simulink model "mech_brownian_osc_control"  (Simulink 7.1)
settings: Solver=ode113  StartTime=0.0  StopTime=300  RelTol=1e-4
PreLoadFcn:
  | % Define primitive constants once
  | 
  | k = 1e-7; b = 12*pi*1e-9; m = 1e-7/16/pi^2; r = 5e-6;
  | kB = 1.3806503e-23; T = 290; g = 2*kB*T*b;
  | lambda = 1e-8; Flambda = 2.5e-12;
InitFcn:
  | % Define system constants once per simulation
  | 
  | brownian.spring.stiffness = k;
  | brownian.spring.damping = b;
  | brownian.spring.offset = 0;
  | 
  | brownian.control.limit = lambda /2;
  | brownian.control.force = Flambda;
  | 
  | brownian.particle.mass = m;
  | brownian.particle.inertia = (2/5)*m*r^2*eye(3);
  | 
  | brownian.noise.power = g;
  | brownian.noise.sample = 2*pi*sqrt(m/k)/100;
  | brownian.noise.seed = 54321;
  | 
  | brownian.dynamics.mintime = 0.01;
  | brownian.dynamics.minlength = sqrt(g/2/b/k)/1000;
libraries: mblibv1 x7, simulink x6
Description:
  | Stochastic Microcontroller
  | 
  | Modified Brownian motion: A microparticle oscillates with a linear damped microspring while diffusing by the addition of a random white noise force. A microcontroller applies a control force that tries to keep the particle within predefined limits.
  | 
  | The system is ergodic: Averages are computed as time averages and assumed to be equal to statistical ensemble averages over long times.  Based on a magnetic microtweezer system for biophysics research.
settings Model: Creator=dkennedy  LastModifiedBy=batserve  ExtModeAutoUpdateStatusClock=off
settings DebuggingCC: SaveWithParameterizedLinksMsg=none  SignalResolutionControl=TryResolveAllWithWarning  SolverPrmCheckMsg=none  MultiTaskDSMMsg=warning  MultiTaskCondExecSysMsg=none
settings HardwareCC: TargetBitPerLong=64  TargetEndianess=LittleEndian  TargetWordSize=64  TargetHWDeviceType=MATLAB Host  ProdEqTarget=off
settings RTWCC: SystemTargetFile=rsim.tlc  TemplateMakefile=rsim_default_tmf  Description=Rapid Simulation Target  ProcessScript=rsim_make_rtw_hook  IncludeERTFirstTime=on
settings RSimTargetCC: TargetFcnLib=ansi_tfl_tmw.mat  TargetFunctionLibrary=ANSI_C  IsPILTarget=off  EnableShiftOperators=on  PortableWordSizes=off

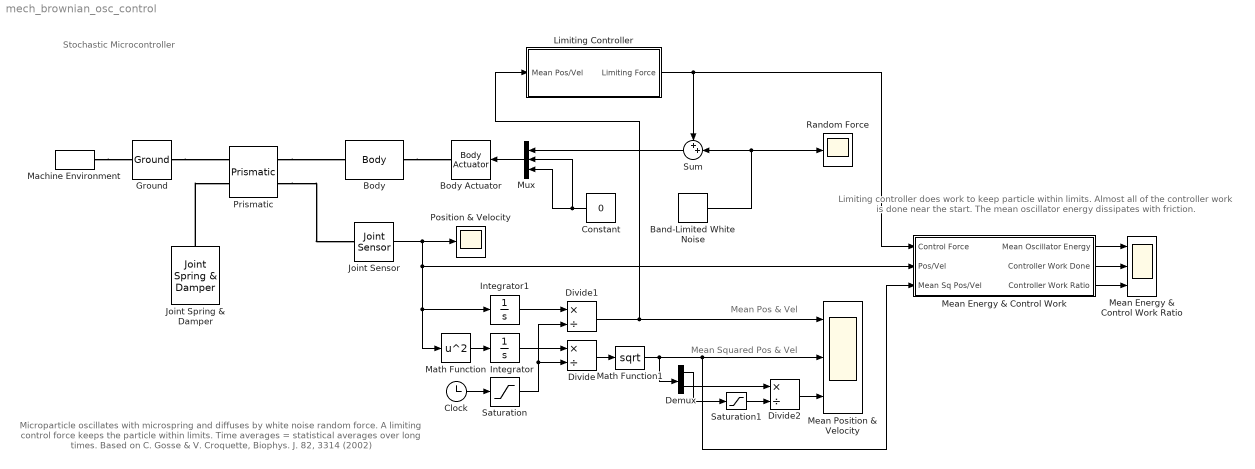
== system mech_brownian_osc_control ==
  note: Mean Pos & Vel
  note: Mean Squared Pos & Vel
  note: Microparticle oscillates with microspring and diffuses by white noise random force.
      | A limiting control force keeps the particle within limits.
      | Time averages = statistical averages over long times.
      | Based on C. Gosse & V. Croquette, Biophys. J. 82, 3314 (2002)
  note: Stochastic Microcontroller
  note: Limiting controller does work to keep particle within limits.
      | Almost all of the controller work is done near the start.
      | The mean oscillator energy dissipates with friction.
  Band-Limited White Noise : simulink/Sources/Band-Limited White Noise  SystemSampleTime=-1  Cov=[brownian.noise.power]  Ts=brownian.noise.sample  seed=brownian.noise.seed
  Body : mblibv1/Bodies/Body  DialogController=MECH.DynMechDlgSource  PhysicalDomain=mechanical  SubClassName=Unknown  LeftPortType=workingframe  RightPortType=workingframe  LConnTagsString=CS1  RConnTagsString=CS2  DialogClass=MechanicalBodyBlock  Mass=brownian.particle.mass  MassUnits=kg  InertiaUnits=kg*m^2  Inertia=brownian.particle.inertia  Shape=Cylinder  ShapeDims=[1 1]  ShapeUnits=m  ShapeUse=false  Density=1  DensityUnits=kg/m^3  DensityUse=false  GraphicsMode=1  BodyColor=[0.5 0.5 0.5]  GraphicsObj=[]  AttachedToCS=1  CG=Left$CG$[0 0 0]$WORLD$WORLD$m$[0 0 0]$Euler X-Y-Z$deg$WORLD$false  WorkingFrames=Left$CS1$[0 0 0]$CG$CG$m$[0 0 0]$Euler X-Y-Z$deg$WORLD$true#Right$CS2$[0 0 0]$CG$CG$m$[0 0 0]$Euler X-Y-Z$deg$WORLD$true  CGPos=[0 0 0]  CGRot=[0 0 0]  CS0Pos=[]  CS0Rot=[]  CS1Pos=[0 0 0]  CS1Rot=[0 0 0]  CS2Pos=[0 0 0]  CS2Rot=[0 0 0]  CS3Pos=[]  CS3Rot=[]  CS4Pos=[]  CS4Rot=[]  CS5Pos=[]  CS5Rot=[]  CS6Pos=[]  CS6Rot=[]  CS7Pos=[]  CS7Rot=[]  CS8Pos=[]  CS8Rot=[]  CS9Pos=[]  CS9Rot=[]  CS10Pos=[]  CS10Rot=[]  CS11Pos=[]  CS11Rot=[]  CS12Pos=[]  CS12Rot=[]  CS13Pos=[]  CS13Rot=[]  CS14Pos=[]  CS14Rot=[]  CS15Pos=[]  CS15Rot=[]  CS16Pos=[]  CS16Rot=[]  CS17Pos=[]  CS17Rot=[]  CS18Pos=[]  CS18Rot=[]  CS19Pos=[]  CS19Rot=[]  CS20Pos=[]  CS20Rot=[]
  Body Actuator : mblibv1/Sensors &  Actuators/Body Actuator  Orientation=left  DialogController=MECH.DynMechDlgSource  SystemSampleTime=-1  PhysicalDomain=Mechanical  PortType=blob  ActuationStyle=Force  AngleUnits=deg  ArcVelocityUnits=deg/s  ArcAccelerationUnits=deg/s^2  CoordPositionUnits=m  VelocityUnits=m/s  AccelerationUnits=m/s^2  ForceUnits=N  TorqueUnits=N*m  ActiveIO=on  Width=3  DialogClass=MechanicalActuatorBlock  ReferenceFrame=Absolute (World)  Angle=off  CoordPosition=on  Force=on  Torque=off
  Clock : Clock
      settings: Decimation=10
  Constant : Constant  Orientation=left  Value=0  OutDataType=sfix(16)  OutScaling=2^0
  Demux : Demux  Outputs=2
  Divide : Product  Inputs=*/  OutDataType=sfix(16)  OutScaling=2^-10
  Divide1 : Product  Inputs=*/  OutDataType=sfix(16)  OutScaling=2^-10
  Divide2 : Product  Inputs=*/  OutDataType=sfix(16)  OutScaling=2^-10
  Ground : mblibv1/Bodies/Ground  DialogController=MECH.DynMechDlgSource  SystemSampleTime=-1  LeftPortType=env  RightPortType=workingframe  PhysicalDomain=Mechanical  DialogClass=GroundBlock  CoordPosition=[0 0 0]  CoordPositionUnits=m  StateVectorMgrId=-1  MachineId=[0 0]  ShowEnvPort=on
  Integrator : Integrator  ZeroCross=off
  Integrator1 : Integrator  ZeroCross=off
  Joint Sensor : mblibv1/Sensors &  Actuators/Joint Sensor  DialogController=MECH.DynMechDlgSource  SystemSampleTime=-1  PhysicalDomain=Mechanical  PortType=blob  Muxed=on  Pose=off  Angle=on  AngleUnits=deg  ArcVelocity=off  ArcVelocityUnits=deg/s  ArcAcceleration=off  ArcAccelerationUnits=deg/s^2  CoordPosition=on  CoordPositionUnits=m  Velocity=on  VelocityUnits=m/s  Acceleration=off  AccelerationUnits=m/s^2  Quaternion=on  QuaternionDT=off  QuaternionDDT=off  QuaternionUnits=off  OutputVector=[1]  ActiveIO=on  Width=2  DialogClass=MechanicalSensorBlock  Primitive=P1  Force=off  ForceUnits=N  Torque=off  TorqueUnits=N*m  ReferenceFrame=Absolute (World)  ReactionSensedSide=Base  ReactionReferenceFrame=Absolute (World)  ReactionForce=off  ReactionForceUnits=N  ReactionMoment=off  ReactionMomentUnits=N*m
  Joint Spring & Damper : mblibv1/Force  Elements/Joint Spring & Damper  Orientation=down  DialogController=MECH.DynMechDlgSource  SystemSampleTime=-1  DialogClass=JointSpringDamper  JFEParameters=P1$true$brownian.spring.stiffness$brownian.spring.damping$brownian.spring.offset$m$m/s$N$deg$deg/s$N-m#P2$false$0$0$0$m$m/s$N$deg$deg/s$N-m#P3$false$0$0$0$m$m/s$N$deg$deg/s$N-m#R1$false$0$0$0$m$m/s$N$deg$deg/s$N-m#R2$false$0$0$0$m$m/s$N$deg$deg/s$N-m#R3$false$0$0$0$m$m/s$N$deg$deg/s$N-m#S$false$0$0$0$m$m/s$N$deg$deg/s$N-m
  Limiting Controller : Subsystem
  Machine Environment : mblibv1/Bodies/Machine Environment  Tag=Factory ground  DialogController=MECH.DialogSource  SystemSampleTime=-1  PortType=env  PhysicalDomain=Mechanical  DialogTemplateClass=MECH.MachineEnvironment  SyncWhenCopied=off  Gravity=[0 -9.81 0]  GravityUnits=m/s^2  GravityAsSignal=off  Dimensionality=Auto-detect  AnalysisType=Forward dynamics  LinearAssemblyTolerance=1e-9  LinearAssemblyToleranceUnits=m  AngularAssemblyTolerance=1e-3  AngularAssemblyToleranceUnits=rad  ConstraintSolverType=Stabilizing  ConstraintRelTolerance=1e-4  ConstraintAbsTolerance=1e-4  UseRobustSingularityHandling=off  RedundancyAnalysisToleranceType=Automatically select tolerance  RedundancyAnalysisTolerance=1e-14  StatePerturbationType=Fixed  PerturbationSize=1e-5  VisualizeMachine=on
  Math Function : Math  Operator=square  OutDataType=sfix(16)  OutScaling=2^0  SaturateOnIntegerOverflow=on
  Math Function1 : Math  Operator=sqrt  OutDataType=sfix(16)  OutScaling=2^0  SaturateOnIntegerOverflow=on
  Mean Energy & Control Work Ratio : Scope  NumInputPorts=3
      settings: TimeRange=300  YMin=0~0~0  YMax=4e-014~5e-016~0.03
  Mean Energy & Control Work : Subsystem
  Mean Position & Velocity : Scope  NumInputPorts=3
      settings: TimeRange=300  YMin=-1e-007~0~0  YMax=1e-007~3e-005~75  SaveName=ScopeData2
  Mux : Mux  Orientation=left  Inputs=3
  Position & Velocity : Scope
      settings: TimeRange=25  YMin=-1e-005  YMax=1e-005  SaveName=ScopeData3
  Prismatic : mblibv1/Joints/Prismatic  DialogController=MECH.DynMechDlgSource  PhysicalDomain=mechanical  SubClassName=Unknown  LeftPortType=blob  RightPortType=blob  LConnTagsString=__newl0|SA1  RConnTagsString=__newr0|SA1  NumSAPorts=2  CutJoint=off  MarkAsCut=off  Primitives=prismatic  PrimitiveProps=P1$World$[1 0 0]$prismatic  DialogClass=JointBlock  P1Axis=[1 0 0]
  Random Force : Scope
      settings: TimeRange=25  YMin=-1e-012  YMax=1e-012
  Saturation : Saturate  UpperLimit=inf  LowerLimit=brownian.dynamics.mintime  ZeroCross=off
  Saturation1 : Saturate  UpperLimit=inf  LowerLimit=brownian.dynamics.minlength  ZeroCross=off
  Sum : Sum  Orientation=left  Inputs=++|  OutDataType=sfix(16)  OutScaling=2^0
  wires:
  Mux/1 -> Body Actuator/1
  Constant/1 -> Mux/3, Mux/2
  Clock/1 -> Saturation/1
  Integrator/1 -> Divide/1
  Math Function/1 -> Integrator/1
  Integrator1/1 -> Divide1/1
  Divide1/1 -> Mean Position & Velocity/1, Limiting Controller/1(Mean Pos/Vel)
  Saturation/1 -> Divide/2, Divide1/2
  Joint Sensor/1 -> Position & Velocity/1, Math Function/1, Integrator1/1, Mean Energy & Control Work/2(Pos/Vel)
  Band-Limited White Noise/1 -> Random Force/1, Sum/2
  Demux/2 -> Divide2/1
  Divide2/1 -> Mean Position & Velocity/3
  Math Function1/1 -> Demux/1, Mean Position & Velocity/2, Mean Energy & Control Work/3(Mean Sq Pos/Vel)
  Divide/1 -> Math Function1/1
  Saturation1/1 -> Divide2/2
  Demux/1 -> Saturation1/1
  Sum/1 -> Mux/1
  Limiting Controller/1(Limiting Force) -> Sum/1, Mean Energy & Control Work/1(Control Force)
  Mean Energy & Control Work/1(Mean Oscillator Energy) -> Mean Energy & Control Work Ratio/1
  Mean Energy & Control Work/2(Controller Work Done) -> Mean Energy & Control Work Ratio/2
  Mean Energy & Control Work/3(Controller Work Ratio) -> Mean Energy & Control Work Ratio/3
  connections:
  Machine Environment/RConn1 -- Ground/LConn1
  Ground/RConn1 -- Prismatic/LConn1
  Prismatic/RConn2 -- Joint Sensor/LConn1
  Body/RConn1 -- Body Actuator/RConn1
  Prismatic/RConn1 -- Body/LConn1
  Joint Spring & Damper/LConn1 -- Prismatic/LConn2

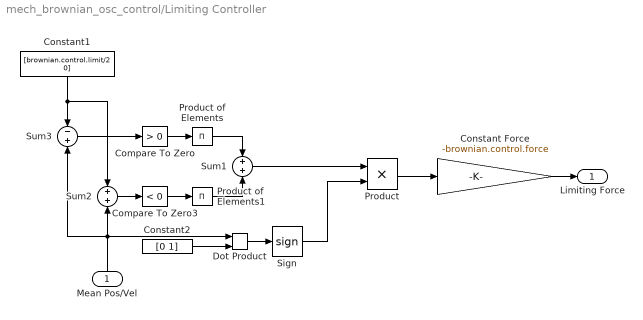
== system mech_brownian_osc_control/Limiting Controller ==
  Mean Pos/Vel : Inport  Orientation=up  OutDataType=sfix(16)  OutScaling=2^0
  Compare To Zero : simulink/Logic and Bit Operations/Compare To Zero  SystemSampleTime=-1  relop=>  LogicOutDataTypeMode=uint8  ZeroCross=off
  Compare To Zero3 : simulink/Logic and Bit Operations/Compare To Zero  SystemSampleTime=-1  relop=<  LogicOutDataTypeMode=uint8  ZeroCross=off
  Constant Force : Gain  Gain=-brownian.control.force  ParameterDataType=sfix(16)  ParameterScaling=2^0  OutDataType=sfix(16)  OutScaling=2^0
  Constant1 : Constant  Orientation=down  Value=[brownian.control.limit/2 0]  OutDataType=sfix(16)  OutScaling=2^0
  Constant2 : Constant  Value=[0 1]  OutDataType=sfix(16)  OutScaling=2^0
  Dot Product : simulink/Math Operations/Dot Product  InputSameDT=on  OutDataType=sfix(16)  OutScaling=2^-10  DoSatur=off
  Product : Product  OutDataType=sfix(16)  OutScaling=2^0  RndMeth=Zero
  Product of Elements : Product  Inputs=1  OutDataType=sfix(16)  OutScaling=2^-10
  Product of Elements1 : Product  Inputs=1  OutDataType=sfix(16)  OutScaling=2^-10
  Sign : Signum  ZeroCross=off
  Sum1 : Sum  OutDataType=sfix(16)  OutScaling=2^0
  Sum2 : Sum  OutDataType=sfix(16)  OutScaling=2^0
  Sum3 : Sum  Inputs=-+  OutDataType=sfix(16)  OutScaling=2^0
  Limiting Force : Outport  OutDataType=sfix(16)  OutScaling=2^0
  wires:
  Constant1/1 -> Sum3/1, Sum2/1
  Constant2/1 -> Dot Product/2
  Dot Product/1 -> Sign/1
  Sum1/1 -> Product/1
  Sign/1 -> Product/2
  Sum3/1 -> Compare To Zero/1
  Compare To Zero/1 -> Product of Elements/1
  Sum2/1 -> Compare To Zero3/1
  Compare To Zero3/1 -> Product of Elements1/1
  Product/1 -> Constant Force/1
  Mean Pos/Vel/1 -> Sum2/2, Sum3/2, Dot Product/1
  Constant Force/1 -> Limiting Force/1
  Product of Elements/1 -> Sum1/1
  Product of Elements1/1 -> Sum1/2

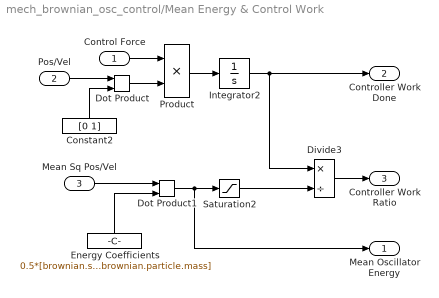
== system mech_brownian_osc_control/Mean Energy & Control Work ==
  Control Force : Inport  OutDataType=sfix(16)  OutScaling=2^0
  Pos/Vel : Inport  Port=2  OutDataType=sfix(16)  OutScaling=2^0
  Mean Sq Pos/Vel : Inport  Port=3  OutDataType=sfix(16)  OutScaling=2^0
  Constant2 : Constant  Orientation=up  Value=[0 1]  OutDataType=sfix(16)  OutScaling=2^0
  Divide3 : Product  Inputs=*/  OutDataType=sfix(16)  OutScaling=2^-10
  Dot Product : simulink/Math Operations/Dot Product  InputSameDT=on  OutDataType=sfix(16)  OutScaling=2^-10  DoSatur=off
  Dot Product1 : simulink/Math Operations/Dot Product  InputSameDT=on  OutDataType=sfix(16)  OutScaling=2^-10  DoSatur=off
  Energy Coefficients : Constant  Orientation=up  Value=0.5*[brownian.spring.stiffness brownian.particle.mass]  OutDataType=sfix(16)  OutScaling=2^0
  Integrator2 : Integrator  ZeroCross=off
  Product : Product  OutDataType=sfix(16)  OutScaling=2^0  RndMeth=Zero
  Saturation2 : Saturate  UpperLimit=inf  LowerLimit=brownian.noise.power/brownian.spring.damping/2  ZeroCross=off
  Mean Oscillator Energy : Outport  OutDataType=sfix(16)  OutScaling=2^0
  Controller Work Done : Outport  Port=2  OutDataType=sfix(16)  OutScaling=2^0
  Controller Work Ratio : Outport  Port=3  OutDataType=sfix(16)  OutScaling=2^0
  wires:
  Constant2/1 -> Dot Product/2
  Dot Product/1 -> Product/2
  Product/1 -> Integrator2/1
  Control Force/1 -> Product/1
  Pos/Vel/1 -> Dot Product/1
  Integrator2/1 -> Divide3/1, Controller Work Done/1
  Mean Sq Pos/Vel/1 -> Dot Product1/1
  Energy Coefficients/1 -> Dot Product1/2
  Dot Product1/1 -> Saturation2/1, Mean Oscillator Energy/1
  Saturation2/1 -> Divide3/2
  Divide3/1 -> Controller Work Ratio/1
